simulink model "MPPT_controll"  (R2018a)
settings: Solver=VariableStepAuto  StartTime=0.0  StopTime=10.0  RelTol=1e-3
values from neighbouring files (symbols this model uses):
  Lambdam = 14.3522    [step2.m]
  Pole = 118    [step2.m]
  R = 58    [step2.m]
  Ro = 1.225    [step2.m]
undefined symbols (not defined in the file or in its folder): Cpmax, Lambda_opt, level, Ls, Ts
libraries: powerlib x4, simulink x2, powerlib_extras x1, simulink_extras x1, peTransforms x1
settings Model: Creator=zxyxi  LastModifiedBy=zxyxi

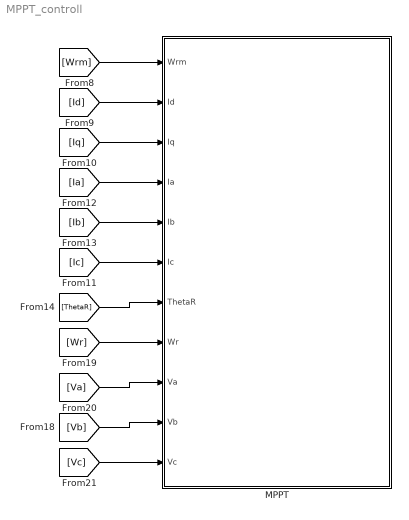
== system MPPT_controll ==
  "MPPT " : Subsystem
  wires:
  [Iq] -> "MPPT "/3("Iq ")
  [Ic] -> "MPPT "/6("Ic ")
  [Vb] -> "MPPT "/10(Vb)
  [Wrm] -> "MPPT "/1(Wrm)
  [Vc] -> "MPPT "/11("Vc ")
  [Va] -> "MPPT "/9(Va)
  [ThetaR] -> "MPPT "/7("ThetaR ")
  [Ib] -> "MPPT "/5("Ib ")
  [Ia] -> "MPPT "/4("Ia ")
  [Id] -> "MPPT "/2("Id ")
  [Wr] -> "MPPT "/8("Wr ")

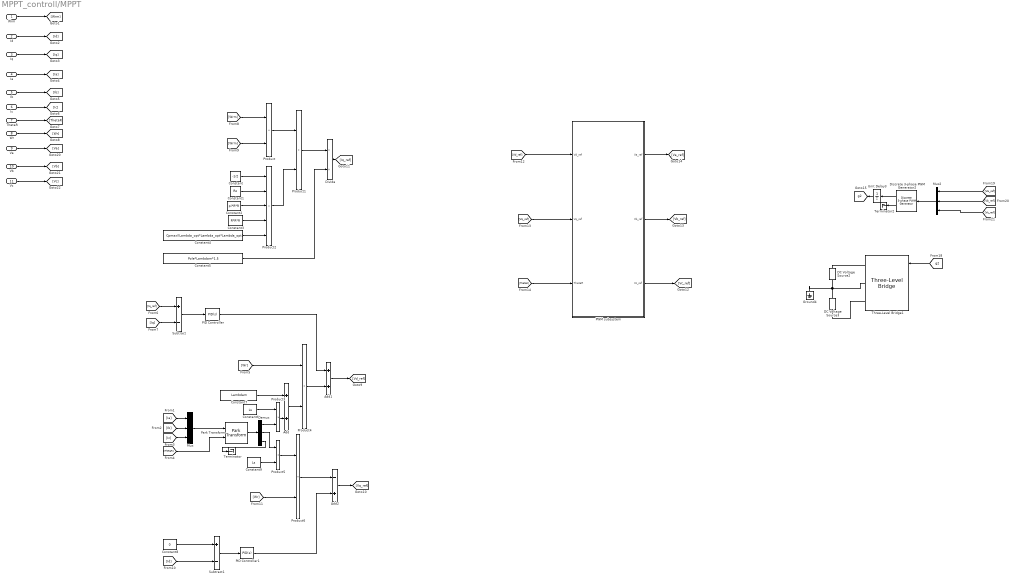
== system MPPT_controll/MPPT  ==
  Wrm : Inport
  "Id " : Inport  Port=2
  "Iq " : Inport  Port=3
  "Ia " : Inport  Port=4
  "Ib " : Inport  Port=5
  "Ic " : Inport  Port=6
  "ThetaR " : Inport  Port=7
  "Wr " : Inport  Port=8
  Va : Inport  Port=9
  Vb : Inport  Port=10
  "Vc " : Inport  Port=11
  Add : Sum
  Add1 : Sum
  Add2 : Sum  Inputs=-+
  Constant : Constant  Value=-1/2
  Constant1 : Constant  Value=Ro
  Constant2 : Constant  Value=pi*R*R
  Constant3 : Constant  Value=R*R*R
  Constant4 : Constant  Value=Cpmax/(Lambda_opt*Lambda_opt*Lambda_opt)
  Constant5 : Constant  Value=Pole*Lambdam*1.5
  Constant6 : Constant  Value=Ls
  Constant7 : Constant  Value=Lambdam
  Constant8 : Constant  Value=0
  Constant9 : Constant  Value=Ls
  DC Voltage Source2 : powerlib/Electrical Sources/DC Voltage Source  Amplitude=2500  Measurements=None
  DC Voltage Source3 : powerlib/Electrical Sources/DC Voltage Source  Amplitude=2500  Measurements=None
  Demux : Demux  Outputs=3
  Discrete 3-phase PWM Generator2 : powerlib_extras/Discrete  Control Blocks/Discrete 3-phase PWM Generator  ModulatorType=3-level  ModulatorMode=Un-synchronized  nF=18  Fc=2400  ModulatingSignals=off  m=0.2  Freq=60  Phase=0  Ts=Ts
  Divide : Product  Inputs=*/
  Ground4 : powerlib/Elements/Ground  LConnTagsString=a
  Mux : Mux  Inputs=3
  Mux2 : Mux  Inputs=3
  PID Controller : simulink/Continuous/PID Controller  Controller=PID  TimeDomain=Continuous-time  SampleTime=-1  IntegratorMethod=Forward Euler  FilterMethod=Forward Euler  Form=Parallel  UseFilter=on  ControllerParametersSource=internal  P=1  I=1  D=0  N=100  InitialConditionSource=internal  InitialConditionForIntegrator=0  InitialConditionForFilter=0  ExternalReset=none  LimitOutput=off  UpperSaturationLimit=inf  LowerSaturationLimit=-inf  LinearizeAsGain=on  AntiWindupMode=none  Kb=1  TrackingMode=off  Kt=1  PParamMin=[]  PParamMax=[]  IParamMin=[]  IParamMax=[]  DParamMin=[]  DParamMax=[]  NParamMin=[]  NParamMax=[]  KbParamMin=[]  KbParamMax=[]  KtParamMin=[]  KtParamMax=[]  POutMin=[]  POutMax=[]  IOutMin=[]  IOutMax=[]  DOutMin=[]  DOutMax=[]  NOutMin=[]  NOutMax=[]  KbOutMin=[]  KbOutMax=[]  KtOutMin=[]  KtOutMax=[]  IntegratorOutMin=[]  IntegratorOutMax=[]  FilterOutMin=[]  FilterOutMax=[]  SumOutMin=[]  SumOutMax=[]  SumI1OutMin=[]  SumI1OutMax=[]  SumI2OutMin=[]  SumI2OutMax=[]  SumI3OutMin=[]  SumI3OutMax=[]  SumDOutMin=[]  SumDOutMax=[]  SaturationOutMin=[]  SaturationOutMax=[]  IntegratorContinuousStateAttributes=''  IntegratorStateMustResolveToSignalObject=off  IntegratorRTWStateStorageClass=Auto  FilterContinuousStateAttributes=''  FilterStateMustResolveToSignalObject=off  FilterRTWStateStorageClass=Auto  DifferentiatorICPrevScaledInput=0  DifferentiatorOutMin=[]  DifferentiatorOutMax=[]  FilterDiffOutCoefMin=[]  FilterDiffOutCoefMax=[]  SumDenOutMin=[]  SumDenOutMax=[]  SumNumOutMin=[]  SumNumOutMax=[]  ReciprocalOutMin=[]  ReciprocalOutMax=[]  DivideOutMin=[]  DivideOutMax=[]  TunerSelectOption=Transfer Function Based (PID Tuner App)
  PID Controller1 : simulink/Continuous/PID Controller  Controller=PID  TimeDomain=Continuous-time  SampleTime=-1  IntegratorMethod=Forward Euler  FilterMethod=Forward Euler  Form=Parallel  UseFilter=on  ControllerParametersSource=internal  P=1  I=1  D=0  N=100  InitialConditionSource=internal  InitialConditionForIntegrator=0  InitialConditionForFilter=0  ExternalReset=none  LimitOutput=off  UpperSaturationLimit=inf  LowerSaturationLimit=-inf  LinearizeAsGain=on  AntiWindupMode=none  Kb=1  TrackingMode=off  Kt=1  PParamMin=[]  PParamMax=[]  IParamMin=[]  IParamMax=[]  DParamMin=[]  DParamMax=[]  NParamMin=[]  NParamMax=[]  KbParamMin=[]  KbParamMax=[]  KtParamMin=[]  KtParamMax=[]  POutMin=[]  POutMax=[]  IOutMin=[]  IOutMax=[]  DOutMin=[]  DOutMax=[]  NOutMin=[]  NOutMax=[]  KbOutMin=[]  KbOutMax=[]  KtOutMin=[]  KtOutMax=[]  IntegratorOutMin=[]  IntegratorOutMax=[]  FilterOutMin=[]  FilterOutMax=[]  SumOutMin=[]  SumOutMax=[]  SumI1OutMin=[]  SumI1OutMax=[]  SumI2OutMin=[]  SumI2OutMax=[]  SumI3OutMin=[]  SumI3OutMax=[]  SumDOutMin=[]  SumDOutMax=[]  SaturationOutMin=[]  SaturationOutMax=[]  IntegratorContinuousStateAttributes=''  IntegratorStateMustResolveToSignalObject=off  IntegratorRTWStateStorageClass=Auto  FilterContinuousStateAttributes=''  FilterStateMustResolveToSignalObject=off  FilterRTWStateStorageClass=Auto  DifferentiatorICPrevScaledInput=0  DifferentiatorOutMin=[]  DifferentiatorOutMax=[]  FilterDiffOutCoefMin=[]  FilterDiffOutCoefMax=[]  SumDenOutMin=[]  SumDenOutMax=[]  SumNumOutMin=[]  SumNumOutMax=[]  ReciprocalOutMin=[]  ReciprocalOutMax=[]  DivideOutMin=[]  DivideOutMax=[]  TunerSelectOption=Transfer Function Based (PID Tuner App)
  "PWM subsystem " : Subsystem
  Park Transform : peTransforms/Park Transform  AxisAlignment=D-axis  PowerInvariant=off
  Product{,1,3..6} (6 alike) : Product
  Product2 : Product  Inputs=5
  Subtract : Sum  Inputs=+-
  Subtract1 : Sum  Inputs=+-
  Terminator : Terminator
  Terminator2 : Terminator
  Three-Level Bridge1 : powerlib/Power Electronics/Three-Level Bridge  Arms=3  SnubberResistance=1e3  SbubberCapacitance=1e-6  Device=Ideal Switches  Ron=0.2e-3  ForwardVoltages="[  2 1 ]"  Measurements=None
      settings: SourceProductName=Simscape Power Systems  SourceProductBaseCode=PS
  Unit Delay3 : UnitDelay  SampleTime=Ts
  tag scope: g2=global
  wires:
  Product2/1 -> Product1/2
  [Wrm] -> Product/2
  Constant5/1 -> Divide/2
  Product1/1 -> Divide/1
  Constant1/1 -> Product2/2
  Constant2/1 -> Product2/3
  Product/1 -> Product1/1
  Divide/1 -> [Iq_ref]
  Constant/1 -> Product2/1
  [Wrm] -> Product/1
  Constant3/1 -> Product2/4
  Constant4/1 -> Product2/5
  Wrm/1 -> [Wrm]
  "Id "/1 -> [Id]
  "Iq "/1 -> [Iq]
  "Ia "/1 -> [Ia]
  "Ib "/1 -> [Ib]
  "Ic "/1 -> [Ic]
  "ThetaR "/1 -> [ThetaR]
  [Ia] -> Mux/1
  [Ic] -> Mux/3
  [Ib] -> Mux/2
  Mux/1 -> Park Transform/1
  [ThetaR] -> Park Transform/2
  Park Transform/1 -> Demux/1
  Demux/1 -> Product3/2
  Constant6/1 -> Product3/1
  Product3/1 -> Add/2
  Constant7/1 -> Add/1
  Add/1 -> Product4/2
  [Wr] -> Product4/1
  "Wr "/1 -> [Wr]
  Product4/1 -> Add1/2
  [Iq_ref] -> Subtract/1
  [Iq] -> Subtract/2
  Subtract/1 -> PID Controller/1
  PID Controller/1 -> Add1/1
  [Id] -> Subtract1/2
  Constant8/1 -> Subtract1/1
  Subtract1/1 -> PID Controller1/1
  Demux/2 -> Product5/1
  Constant9/1 -> Product5/2
  Product5/1 -> Product6/1
  [Wr] -> Product6/2
  Product6/1 -> Add2/1
  PID Controller1/1 -> Add2/2
  Add1/1 -> [Vd_ref]
  Add2/1 -> [Vq_ref]
  Vb/1 -> [Vb]
  "Vc "/1 -> [Vc]
  Va/1 -> [Va]
  [Vd_ref] -> "PWM subsystem "/1("Vd_ref ")
  [Vq_ref] -> "PWM subsystem "/2("Vq_ref ")
  [ThetaR] -> "PWM subsystem "/3("ThetaR ")
  "PWM subsystem "/3("Vc_ref ") -> [Vc_ref]
  "PWM subsystem "/2("Vb_ref ") -> [Vb_ref]
  "PWM subsystem "/1("Va_ref ") -> [Va_ref]
  Demux/3 -> Terminator/1
  Discrete 3-phase PWM Generator2/2 -> Terminator2/1
  Discrete 3-phase PWM Generator2/1 -> Unit Delay3/1
  Mux2/1 -> Discrete 3-phase PWM Generator2/1
  Unit Delay3/1 -> [g2]
  [Va_ref] -> Mux2/1
  [Vb_ref] -> Mux2/2
  [Vc_ref] -> Mux2/3
  [g2] -> Three-Level Bridge1/1
  connections:
  Three-Level Bridge1/RConn1 -- DC Voltage Source2/RConn1
  Three-Level Bridge1/RConn3 -- DC Voltage Source3/LConn1
  DC Voltage Source3/RConn1 -- Ground4/LConn1 -- Three-Level Bridge1/RConn2 -- DC Voltage Source2/LConn1

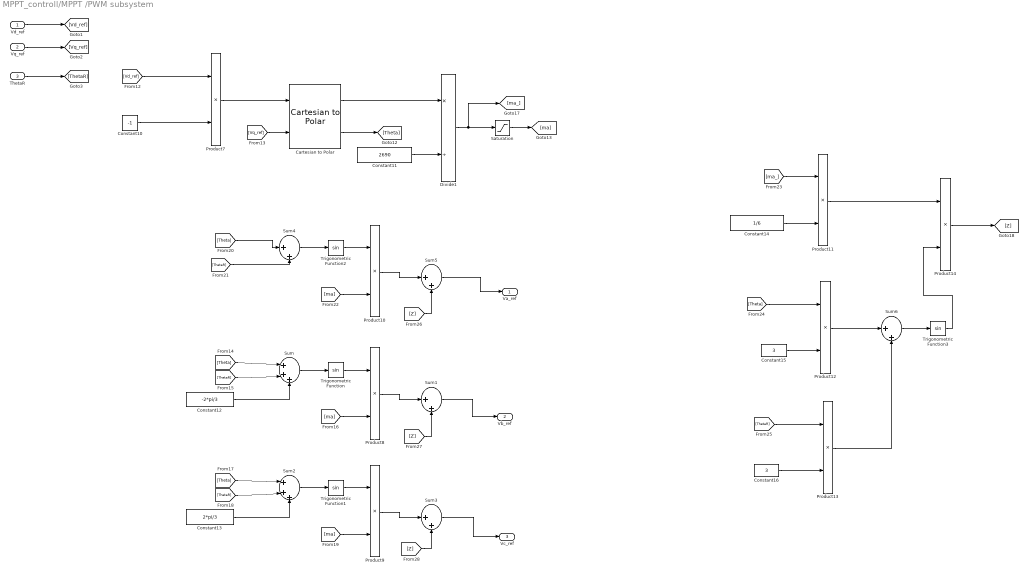
== system MPPT_controll/MPPT /PWM subsystem  ==
  "Vd_ref " : Inport
  "Vq_ref " : Inport  Port=2
  "ThetaR " : Inport  Port=3
  Cartesian to Polar : simulink_extras/Transformations/Cartesian to Polar
      settings: SourceProductName=Simulink
  Constant10 : Constant  Value=-1
  Constant11 : Constant  Value=2690
  Constant12 : Constant  Value=-2*pi/3
  Constant13 : Constant  Value=2*pi/3
  Constant14 : Constant  Value=1/6
  Constant15 : Constant  Value=3
  Constant16 : Constant  Value=3
  Divide1 : Product  Inputs=*/
  Product{7..14} (8 alike) : Product
  Saturation : Saturate  UpperLimit=1  LowerLimit=0
  Sum : Sum  Inputs=|+++
  Sum{1,3..6} (5 alike) : Sum  Inputs=|++
  Sum2 : Sum  Inputs=|+++
  Trigonometric Function{,1..3} (4 alike) : Trigonometry
  "Va_ref " : Outport
  "Vb_ref " : Outport  Port=2
  "Vc_ref " : Outport  Port=3
  wires:
  [Z] -> Sum3/2
  [Vq_ref] -> Cartesian to Polar/2
  [ma_] -> Product11/1
  [ThetaR] -> Sum/2
  Constant12/1 -> Sum/3
  Product10/1 -> Sum5/1
  [Vd_ref] -> Product7/1
  [ThetaR] -> Product13/1
  Product7/1 -> Cartesian to Polar/1
  [Theta] -> Product12/1
  Sum2/1 -> Trigonometric Function1/1
  [Theta] -> Sum/1
  [ma] -> Product9/2
  Cartesian to Polar/1 -> Divide1/1
  [ma] -> Product8/2
  Product13/1 -> Sum6/2
  Sum6/1 -> Trigonometric Function3/1
  Constant13/1 -> Sum2/3
  [Z] -> Sum1/2
  Constant15/1 -> Product12/2
  Constant16/1 -> Product13/2
  Product9/1 -> Sum3/1
  Saturation/1 -> [ma]
  Trigonometric Function2/1 -> Product10/1
  Divide1/1 -> [ma_], Saturation/1
  Cartesian to Polar/2 -> [Theta]
  Sum/1 -> Trigonometric Function/1
  Product12/1 -> Sum6/1
  Product14/1 -> [Z]
  Trigonometric Function3/1 -> Product14/2
  Constant14/1 -> Product11/2
  [Z] -> Sum5/2
  Constant11/1 -> Divide1/2
  Sum3/1 -> "Vc_ref "/1
  Trigonometric Function1/1 -> Product9/1
  [Theta] -> Sum2/1
  [ThetaR] -> Sum2/2
  Product11/1 -> Product14/1
  Sum4/1 -> Trigonometric Function2/1
  Sum5/1 -> "Va_ref "/1
  [ThetaR] -> Sum4/2
  Constant10/1 -> Product7/2
  [Theta] -> Sum4/1
  [ma] -> Product10/2
  Sum1/1 -> "Vb_ref "/1
  Trigonometric Function/1 -> Product8/1
  Product8/1 -> Sum1/1
  "Vd_ref "/1 -> [Vd_ref]
  "Vq_ref "/1 -> [Vq_ref]
  "ThetaR "/1 -> [ThetaR]
